simulink model "Vehicle_trailer"  (R2015a)
settings: Solver=ode3  StartTime=0.0  StopTime=30.0  FixedStep=0.2  RelTol=1e-3
undefined symbols (not defined in the file): L1, L12, L2, v
settings Model: Creator=Sara  LastModifiedBy=Sara

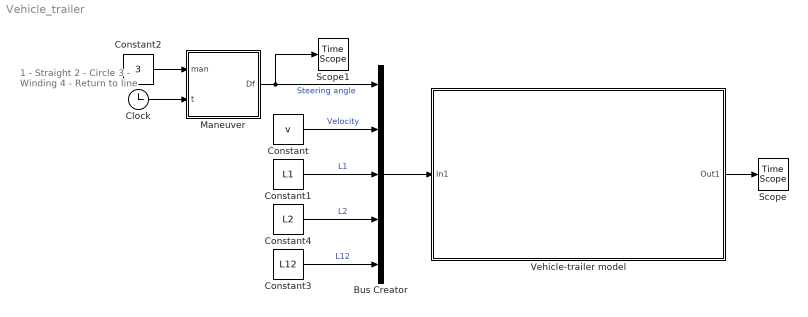
== system Vehicle_trailer ==
  note: 1 - Straight
      | 2 - Circle
      | 3 - Winding
      | 4 - Return to line
  Bus Creator : BusCreator  Inputs=5
  Clock : Clock
  Constant : Constant  Value=v
  Constant1 : Constant  Value=L1
  Constant2 : Constant  Value=3
  Constant3 : Constant  Value=L12
  Constant4 : Constant  Value=L2
  Maneuver : MATLAB Function  TreatAsAtomicUnit=on
  Scope : TimeScope
  Scope1 : TimeScope
  Vehicle-trailer model : Subsystem
      mask Display: image(imread('vt.png'))
  wires:
  Constant/1 -> Bus Creator/2  "Velocity"
  Constant1/1 -> Bus Creator/3  "L1"
  Constant4/1 -> Bus Creator/4  "L2"
  Constant3/1 -> Bus Creator/5  "L12"
  Bus Creator/1 -> Vehicle-trailer model/1(In1)
  Maneuver/1(Df) -> Scope1/1, Bus Creator/1  "Steering angle"
  Constant2/1 -> Maneuver/1(man)
  Clock/1 -> Maneuver/2(t)
  Vehicle-trailer model/1(Out1) -> Scope/1

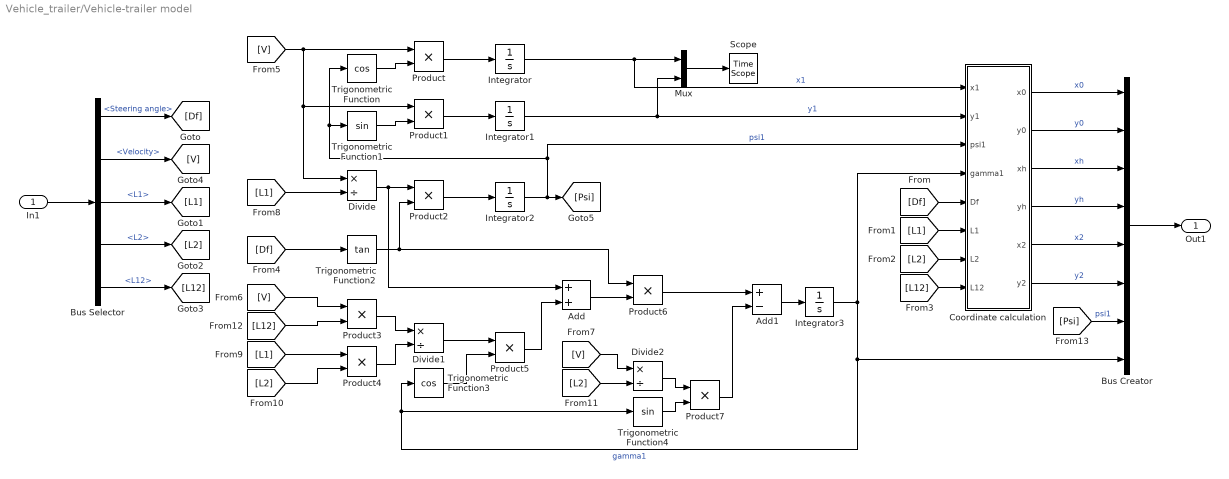
== system Vehicle_trailer/Vehicle-trailer model ==
  In1 : Inport
  Add : Sum
  Add1 : Sum  Inputs=+-
  Bus Creator : BusCreator  Inputs=8
  Bus Selector : BusSelector  OutputSignals=Steering angle,Velocity,L1,L2,L12
  Coordinate calculation : MATLAB Function  TreatAsAtomicUnit=on
  Divide : Product  Inputs=*/
  Divide1 : Product  Inputs=*/
  Divide2 : Product  Inputs=*/
  Integrator{,1..3} (4 alike) : Integrator
  Mux : Mux  Inputs=2
  Product{,1..7} (8 alike) : Product
  Scope : TimeScope
  Trigonometric Function : Trigonometry  Operator=cos
  Trigonometric Function1 : Trigonometry
  Trigonometric Function2 : Trigonometry  Operator=tan
  Trigonometric Function3 : Trigonometry  Operator=cos
  Trigonometric Function4 : Trigonometry
  Out1 : Outport
  wires:
  Trigonometric Function4/1 -> Product7/2
  Divide2/1 -> Product7/1
  Trigonometric Function1/1 -> Product1/2
  Product1/1 -> Integrator1/1
  In1/1 -> Bus Selector/1
  Trigonometric Function3/1 -> Product5/2
  Product2/1 -> Integrator2/1
  Divide/1 -> Product2/1, Add/1
  Trigonometric Function2/1 -> Product6/1, Product2/2
  Product6/1 -> Add1/1
  Add1/1 -> Integrator3/1
  Divide1/1 -> Product5/1
  Integrator3/1 -> Bus Creator/8, Trigonometric Function4/1, Trigonometric Function3/1, Coordinate calculation/4(gamma1)  "gamma1"
  Product7/1 -> Add1/2
  Add/1 -> Product6/2
  Product3/1 -> Divide1/1
  Integrator2/1 -> [Psi], Trigonometric Function/1, Trigonometric Function1/1, Coordinate calculation/3(psi1)  "psi1"
  Trigonometric Function/1 -> Product/2
  Product5/1 -> Add/2
  Product4/1 -> Divide1/2
  Product/1 -> Integrator/1
  Bus Selector/1 -> [Df]  "<Steering angle>"
  Bus Selector/5 -> [L12]  "<L12>"
  Bus Selector/3 -> [L1]  "<L1>"
  Bus Selector/4 -> [L2]  "<L2>"
  Integrator/1 -> Coordinate calculation/1(x1), Mux/1  "x1"
  Integrator1/1 -> Mux/2, Coordinate calculation/2(y1)  "y1"
  Mux/1 -> Scope/1
  Bus Creator/1 -> Out1/1
  [Df] -> Coordinate calculation/5(Df)
  [L1] -> Coordinate calculation/6(L1)
  [L2] -> Coordinate calculation/7(L2)
  [L12] -> Coordinate calculation/8(L12)
  [Df] -> Trigonometric Function2/1
  Bus Selector/2 -> [V]  "<Velocity>"
  [V] -> Divide/1, Product1/1, Product/1
  [V] -> Product3/1
  [V] -> Divide2/1
  [L1] -> Divide/2
  [L1] -> Product4/1
  [L2] -> Product4/2
  [L2] -> Divide2/2
  [L12] -> Product3/2
  Coordinate calculation/1(x0) -> Bus Creator/1  "x0"
  Coordinate calculation/2(y0) -> Bus Creator/2  "y0"
  [Psi] -> Bus Creator/7  "psi1"
  Coordinate calculation/3(xh) -> Bus Creator/3  "xh"
  Coordinate calculation/4(yh) -> Bus Creator/4  "yh"
  Coordinate calculation/5(x2) -> Bus Creator/5  "x2"
  Coordinate calculation/6(y2) -> Bus Creator/6  "y2"

== matlab function Vehicle_trailer/Maneuver ==
  data: man input; Df output; t input
function Df = fcn(man,t)
switch man
    case 1
        Df=0;
    case 2
        Df=0.26;
    case 3
        if t<5
            Df=0;
        elseif (t>=5) && (t<10)
            Df=0.26;
        elseif (t>=10) && (t<15)
            Df=0;
        elseif (t>=15) && (t<20)
            Df=-0.26;
        elseif (t>=20) && (t<25)
            Df=0;
        else
            Df=0.26;
        end
    case 4
        if t<5
            Df=0;
        elseif (t>=5) && (t<10)
            Df=0.7;
        else
            Df=0;
        end
    otherwise
        Df=0;
end

== matlab function Vehicle_trailer/Vehicle-trailer model/Coordinate calculation ==
  data: x1 input; x0 output; y1 input; psi1 input; gamma1 input; Df input; L1 input; L2 input; L12 input; y0 output; xh output; yh output; x2 output; y2 output
function [x0,y0,xh,yh,x2,y2] = fcn(x1,y1,psi1,gamma1,Df,L1,L2,L12)
psi2=psi1-gamma1;
psi0=psi1+Df;

x0=x1+L1*cos(psi1);
y0=y1+L1*sin(psi1);
xh=x1-L12*cos(psi1);
yh=y1-L12*sin(psi1);
x2=x1-L12*cos(psi1)-L2*cos(psi2);
y2=y1-L12*sin(psi1)-L2*sin(psi2);
